simulink subsystem "DirectCommands"  (R2021b)
settings: Solver=VariableStepAuto  StartTime=0.0  StopTime=10.0  RelTol=1e-3
libraries: mbdriLib x1
settings Model: Creator=promero  LastModifiedBy=promero

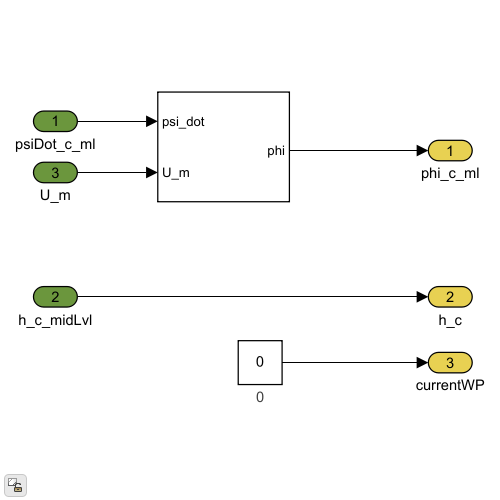
[thumbnail: Simulink's stored preview of the top-level diagram]
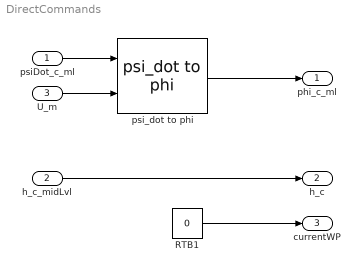
== system DirectCommands ==
  psiDot_c_ml : Inport
  h_c_midLvl : Inport  Port=2
  U_m : Inport  Port=3
  RTB1 : Constant  Value=0  OutDataTypeStr=uint8
      settings: AttributesFormatString=%<Value>
  psi_dot to phi : mbdriLib/Angles and Units/psi_dot to phi  SystemSampleTime=-1  VariantActivationTime=update diagram  Latency=0  AutoFrameSizeCalculation=off
  phi_c_ml : Outport  VectorParamsAs1DForOutWhenUnconnected=off
  h_c : Outport  Port=2  VectorParamsAs1DForOutWhenUnconnected=off
  currentWP : Outport  Port=3  VectorParamsAs1DForOutWhenUnconnected=off
  wires:
  psiDot_c_ml/1 -> psi_dot to phi/1
  psi_dot to phi/1 -> phi_c_ml/1
  RTB1/1 -> currentWP/1
  U_m/1 -> psi_dot to phi/2
  h_c_midLvl/1 -> h_c/1
